simulink model "test_mdl_NI"  (R2018a)
settings: Solver=VariableStepAuto  StartTime=0.0  StopTime=10.0  RelTol=1e-3
(part 4 of 24)

== system test_mdl_NI/CAN_Signal/ABS_ESC/TesterPhysicalResABS_0x768 ==
  in : Inport
  TesterPhysicalResABS : Subsystem
  bus_creator : BusCreator  Inputs=1
  bus_selector : BusSelector  OutputSignals=TesterPhysicalResABS
  out_port : Outport
  wires:
  bus_creator/1 -> out_port/1  "TesterPhysicalResABS_0x768"
  TesterPhysicalResABS/1(out) -> bus_creator/1  "TesterPhysicalResABS"
  bus_selector/1 -> TesterPhysicalResABS/1(in)  "<TesterPhysicalResABS>"
  in/1 -> bus_selector/1

== system test_mdl_NI/CAN_Signal/ABS_ESC/TrailerBrakeData_0x412 ==
  in : Inport
  TrlrBrk_Pc_Rq : Subsystem
  VehPtch_An_Dsply : Subsystem
  VehRol_An_Dsply : Subsystem
  bus_creator : BusCreator  Inputs=3
  bus_selector : BusSelector  OutputSignals=TrlrBrk_Pc_Rq,VehPtch_An_Dsply,VehRol_An_Dsply
  out_port : Outport
  wires:
  bus_creator/1 -> out_port/1  "TrailerBrakeData_0x412"
  TrlrBrk_Pc_Rq/1(out) -> bus_creator/1  "TrlrBrk_Pc_Rq"
  VehPtch_An_Dsply/1(out) -> bus_creator/2  "VehPtch_An_Dsply"
  VehRol_An_Dsply/1(out) -> bus_creator/3  "VehRol_An_Dsply"
  bus_selector/1 -> TrlrBrk_Pc_Rq/1(in)  "<TrlrBrk_Pc_Rq>"
  bus_selector/2 -> VehPtch_An_Dsply/1(in)  "<VehPtch_An_Dsply>"
  bus_selector/3 -> VehRol_An_Dsply/1(in)  "<VehRol_An_Dsply>"
  in/1 -> bus_selector/1

== system test_mdl_NI/CAN_Signal/ABS_ESC/WheelData_0x216 ==
  in : Inport
  BrkObdData_No_Actl : Subsystem
  BrkObdIndex_No_Actl : Subsystem
  WhlDirFl_D_Actl : Subsystem
  WhlDirFr_D_Actl : Subsystem
  WhlDirRl_D_Actl : Subsystem
  WhlDirRr_D_Actl : Subsystem
  WhlRotatFl_No_Cnt : Subsystem
  WhlRotatFr_No_Cnt : Subsystem
  WhlRotatRl_No_Cnt : Subsystem
  WhlRotatRr_No_Cnt : Subsystem
  bus_creator : BusCreator  Inputs=10
  bus_selector : BusSelector  OutputSignals=WhlRotatFr_No_Cnt,WhlRotatFl_No_Cnt,WhlRotatRr_No_Cnt,WhlRotatRl_No_Cnt,WhlDirRl_D_Actl,WhlDirFr_D_Actl,WhlDirFl_D_Actl,WhlDirRr_D_Actl,BrkObdIndex_No_Actl,BrkObdData_No_Actl
  out_port : Outport
  wires:
  bus_creator/1 -> out_port/1  "WheelData_0x216"
  WhlRotatFr_No_Cnt/1(out) -> bus_creator/1  "WhlRotatFr_No_Cnt"
  WhlRotatFl_No_Cnt/1(out) -> bus_creator/2  "WhlRotatFl_No_Cnt"
  WhlRotatRr_No_Cnt/1(out) -> bus_creator/3  "WhlRotatRr_No_Cnt"
  WhlRotatRl_No_Cnt/1(out) -> bus_creator/4  "WhlRotatRl_No_Cnt"
  WhlDirRl_D_Actl/1(out) -> bus_creator/5  "WhlDirRl_D_Actl"
  WhlDirFr_D_Actl/1(out) -> bus_creator/6  "WhlDirFr_D_Actl"
  WhlDirFl_D_Actl/1(out) -> bus_creator/7  "WhlDirFl_D_Actl"
  WhlDirRr_D_Actl/1(out) -> bus_creator/8  "WhlDirRr_D_Actl"
  BrkObdIndex_No_Actl/1(out) -> bus_creator/9  "BrkObdIndex_No_Actl"
  BrkObdData_No_Actl/1(out) -> bus_creator/10  "BrkObdData_No_Actl"
  bus_selector/1 -> WhlRotatFr_No_Cnt/1(in)  "<WhlRotatFr_No_Cnt>"
  bus_selector/2 -> WhlRotatFl_No_Cnt/1(in)  "<WhlRotatFl_No_Cnt>"
  bus_selector/3 -> WhlRotatRr_No_Cnt/1(in)  "<WhlRotatRr_No_Cnt>"
  bus_selector/4 -> WhlRotatRl_No_Cnt/1(in)  "<WhlRotatRl_No_Cnt>"
  bus_selector/5 -> WhlDirRl_D_Actl/1(in)  "<WhlDirRl_D_Actl>"
  bus_selector/6 -> WhlDirFr_D_Actl/1(in)  "<WhlDirFr_D_Actl>"
  bus_selector/7 -> WhlDirFl_D_Actl/1(in)  "<WhlDirFl_D_Actl>"
  bus_selector/8 -> WhlDirRr_D_Actl/1(in)  "<WhlDirRr_D_Actl>"
  bus_selector/9 -> BrkObdIndex_No_Actl/1(in)  "<BrkObdIndex_No_Actl>"
  bus_selector/10 -> BrkObdData_No_Actl/1(in)  "<BrkObdData_No_Actl>"
  in/1 -> bus_selector/1

== system test_mdl_NI/CAN_Signal/ABS_ESC/WheelSpeed_0x217 ==
  in : Inport
  WhlFl_W_Meas : Subsystem
  WhlFr_W_Meas : Subsystem
  WhlRl_W_Meas : Subsystem
  WhlRr_W_Meas : Subsystem
  bus_creator : BusCreator  Inputs=4
  bus_selector : BusSelector  OutputSignals=WhlFl_W_Meas,WhlFr_W_Meas,WhlRl_W_Meas,WhlRr_W_Meas
  out_port : Outport
  wires:
  bus_creator/1 -> out_port/1  "WheelSpeed_0x217"
  WhlFl_W_Meas/1(out) -> bus_creator/1  "WhlFl_W_Meas"
  WhlFr_W_Meas/1(out) -> bus_creator/2  "WhlFr_W_Meas"
  WhlRl_W_Meas/1(out) -> bus_creator/3  "WhlRl_W_Meas"
  WhlRr_W_Meas/1(out) -> bus_creator/4  "WhlRr_W_Meas"
  bus_selector/1 -> WhlFl_W_Meas/1(in)  "<WhlFl_W_Meas>"
  bus_selector/2 -> WhlFr_W_Meas/1(in)  "<WhlFr_W_Meas>"
  bus_selector/3 -> WhlRl_W_Meas/1(in)  "<WhlRl_W_Meas>"
  bus_selector/4 -> WhlRr_W_Meas/1(in)  "<WhlRr_W_Meas>"
  in/1 -> bus_selector/1

== system test_mdl_NI/CAN_Signal/ADAS/ACCDATA ==
  in : Inport
  AccBrkDecel_B_Rq : Subsystem
  AccBrkPrchg_B_Rq : Subsystem
  AccBrkTot_A_Rq : Subsystem
  AccCancl_B_Rq : Subsystem
  AccPrpl_A_Rq : Subsystem
  AccPrpl_A_Rq1 : Subsystem
  AccStopStat_B_Rq : Subsystem
  CmbbEngTqMn_B_Rq : Subsystem
  bus_creator : BusCreator  Inputs=8
  bus_selector : BusSelector  OutputSignals=AccBrkPrchg_B_Rq,AccBrkDecel_B_Rq,AccStopStat_B_Rq,AccBrkTot_A_Rq,CmbbEngTqMn_B_Rq,AccCancl_B_Rq,AccPrpl_A_Rq,AccPrpl_A_Rq1
  out_port : Outport
  wires:
  bus_creator/1 -> out_port/1  "ACCDATA"
  AccBrkPrchg_B_Rq/1(out) -> bus_creator/1  "AccBrkPrchg_B_Rq"
  AccBrkDecel_B_Rq/1(out) -> bus_creator/2  "AccBrkDecel_B_Rq"
  AccStopStat_B_Rq/1(out) -> bus_creator/3  "AccStopStat_B_Rq"
  AccBrkTot_A_Rq/1(out) -> bus_creator/4  "AccBrkTot_A_Rq"
  CmbbEngTqMn_B_Rq/1(out) -> bus_creator/5  "CmbbEngTqMn_B_Rq"
  AccCancl_B_Rq/1(out) -> bus_creator/6  "AccCancl_B_Rq"
  AccPrpl_A_Rq/1(out) -> bus_creator/7  "AccPrpl_A_Rq"
  AccPrpl_A_Rq1/1(out) -> bus_creator/8  "AccPrpl_A_Rq1"
  bus_selector/1 -> AccBrkPrchg_B_Rq/1(in)  "<AccBrkPrchg_B_Rq>"
  bus_selector/2 -> AccBrkDecel_B_Rq/1(in)  "<AccBrkDecel_B_Rq>"
  bus_selector/3 -> AccStopStat_B_Rq/1(in)  "<AccStopStat_B_Rq>"
  bus_selector/4 -> AccBrkTot_A_Rq/1(in)  "<AccBrkTot_A_Rq>"
  bus_selector/5 -> CmbbEngTqMn_B_Rq/1(in)  "<CmbbEngTqMn_B_Rq>"
  bus_selector/6 -> AccCancl_B_Rq/1(in)  "<AccCancl_B_Rq>"
  bus_selector/7 -> AccPrpl_A_Rq/1(in)  "<AccPrpl_A_Rq>"
  bus_selector/8 -> AccPrpl_A_Rq1/1(in)  "<AccPrpl_A_Rq1>"
  in/1 -> bus_selector/1

== system test_mdl_NI/CAN_Signal/ADAS/ACCDATA_2 ==
  in : Inport
  CmbbBaSens_D_Rq : Subsystem
  CmbbBrkDecel_A_Rq : Subsystem
  CmbbBrkDecel_B_Rq : Subsystem
  CmbbBrkPrchg_D_Rq : Subsystem
  bus_creator : BusCreator  Inputs=4
  bus_selector : BusSelector  OutputSignals=CmbbBrkPrchg_D_Rq,CmbbBrkDecel_A_Rq,CmbbBaSens_D_Rq,CmbbBrkDecel_B_Rq
  out_port : Outport
  wires:
  bus_creator/1 -> out_port/1  "ACCDATA_2"
  CmbbBrkPrchg_D_Rq/1(out) -> bus_creator/1  "CmbbBrkPrchg_D_Rq"
  CmbbBrkDecel_A_Rq/1(out) -> bus_creator/2  "CmbbBrkDecel_A_Rq"
  CmbbBaSens_D_Rq/1(out) -> bus_creator/3  "CmbbBaSens_D_Rq"
  CmbbBrkDecel_B_Rq/1(out) -> bus_creator/4  "CmbbBrkDecel_B_Rq"
  bus_selector/1 -> CmbbBrkPrchg_D_Rq/1(in)  "<CmbbBrkPrchg_D_Rq>"
  bus_selector/2 -> CmbbBrkDecel_A_Rq/1(in)  "<CmbbBrkDecel_A_Rq>"
  bus_selector/3 -> CmbbBaSens_D_Rq/1(in)  "<CmbbBaSens_D_Rq>"
  bus_selector/4 -> CmbbBrkDecel_B_Rq/1(in)  "<CmbbBrkDecel_B_Rq>"
  in/1 -> bus_selector/1

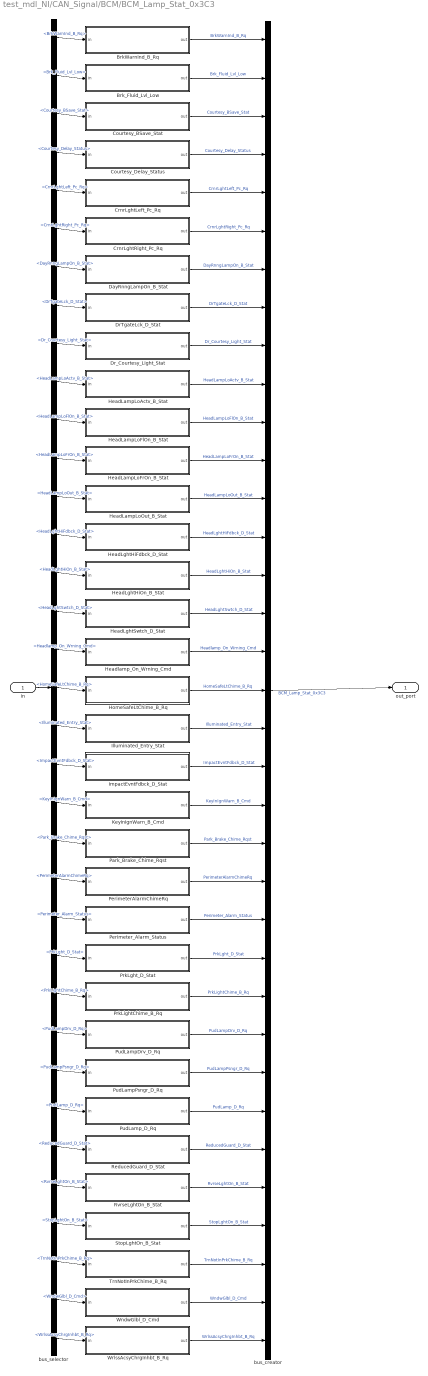
== system test_mdl_NI/CAN_Signal/BCM/BCM_Lamp_Stat_0x3C3 ==
  in : Inport
  BrkWarnInd_B_Rq : Subsystem
  Brk_Fluid_Lvl_Low : Subsystem
  Courtesy_BSave_Stat : Subsystem
  Courtesy_Delay_Status : Subsystem
  CrnrLghtLeft_Pc_Rq : Subsystem
  CrnrLghtRight_Pc_Rq : Subsystem
  DayRnngLampOn_B_Stat : Subsystem
  DrTgateLck_D_Stat : Subsystem
  Dr_Courtesy_Light_Stat : Subsystem
  HeadLampLoActv_B_Stat : Subsystem
  HeadLampLoFlOn_B_Stat : Subsystem
  HeadLampLoFrOn_B_Stat : Subsystem
  HeadLampLoOut_B_Stat : Subsystem
  HeadLghtHiFdbck_D_Stat : Subsystem
  HeadLghtHiOn_B_Stat : Subsystem
  HeadLghtSwtch_D_Stat : Subsystem
  Headlamp_On_Wrning_Cmd : Subsystem
  HomeSafeLtChime_B_Rq : Subsystem
  Illuminated_Entry_Stat : Subsystem
  ImpactEvntFdbck_D_Stat : Subsystem
  KeyInIgnWarn_B_Cmd : Subsystem
  Park_Brake_Chime_Rqst : Subsystem
  PerimeterAlarmChimeRq : Subsystem
  Perimeter_Alarm_Status : Subsystem
  PrkLght_D_Stat : Subsystem
  PrkLightChime_B_Rq : Subsystem
  PudLampDrv_D_Rq : Subsystem
  PudLampPsngr_D_Rq : Subsystem
  PudLamp_D_Rq : Subsystem
  ReducedGuard_D_Stat : Subsystem
  RvrseLghtOn_B_Stat : Subsystem
  StopLghtOn_B_Stat : Subsystem
  TrnNotInPrkChime_B_Rq : Subsystem
  WndwGlbl_D_Cmd : Subsystem
  WrlssAcsyChrgInhbt_B_Rq : Subsystem
  bus_creator : BusCreator  Inputs=35
  bus_selector : BusSelector  OutputSignals=BrkWarnInd_B_Rq,Brk_Fluid_Lvl_Low,Courtesy_BSave_Stat,Courtesy_Delay_Status,CrnrLghtLeft_Pc_Rq,CrnrLghtRight_Pc_Rq,DayRnngLampOn_B_Stat,DrTgateLck_D_Stat,Dr_Courtesy_Light_Stat,HeadLampLoActv_B_Stat,HeadLampLoFlOn_B_Stat,HeadLampLoFrOn_B_Stat,HeadLampLoOut_B_Stat,HeadLghtHiFdbck_D_Stat,HeadLghtHiOn_B_Stat,HeadLghtSwtch_D_Stat,Headlamp_On_Wrning_Cmd,HomeSafeLtChime_B_Rq,Illuminated_Entry_Stat,ImpactEvntFdbck_D_Stat,KeyInIgnWarn_B_Cmd,Park_Brake_Chime_Rqst,PerimeterAlarmChimeRq,Perimeter_Alarm_Status,PrkLght_D_Stat,PrkLightChime_B_Rq,PudLampDrv_D_Rq,PudLampPsngr_D_Rq,PudLamp_D_Rq,ReducedGuard_D_Stat,RvrseLghtOn_B_Stat,StopLghtOn_B_Stat,TrnNotInPrkChime_B_Rq,WndwGlbl_D_Cmd,WrlssAcsyChrgInhbt_B_Rq
  out_port : Outport
  wires:
  bus_creator/1 -> out_port/1  "BCM_Lamp_Stat_0x3C3"
  BrkWarnInd_B_Rq/1(out) -> bus_creator/1  "BrkWarnInd_B_Rq"
  Brk_Fluid_Lvl_Low/1(out) -> bus_creator/2  "Brk_Fluid_Lvl_Low"
  Courtesy_BSave_Stat/1(out) -> bus_creator/3  "Courtesy_BSave_Stat"
  Courtesy_Delay_Status/1(out) -> bus_creator/4  "Courtesy_Delay_Status"
  CrnrLghtLeft_Pc_Rq/1(out) -> bus_creator/5  "CrnrLghtLeft_Pc_Rq"
  CrnrLghtRight_Pc_Rq/1(out) -> bus_creator/6  "CrnrLghtRight_Pc_Rq"
  DayRnngLampOn_B_Stat/1(out) -> bus_creator/7  "DayRnngLampOn_B_Stat"
  DrTgateLck_D_Stat/1(out) -> bus_creator/8  "DrTgateLck_D_Stat"
  Dr_Courtesy_Light_Stat/1(out) -> bus_creator/9  "Dr_Courtesy_Light_Stat"
  HeadLampLoActv_B_Stat/1(out) -> bus_creator/10  "HeadLampLoActv_B_Stat"
  HeadLampLoFlOn_B_Stat/1(out) -> bus_creator/11  "HeadLampLoFlOn_B_Stat"
  HeadLampLoFrOn_B_Stat/1(out) -> bus_creator/12  "HeadLampLoFrOn_B_Stat"
  HeadLampLoOut_B_Stat/1(out) -> bus_creator/13  "HeadLampLoOut_B_Stat"
  HeadLghtHiFdbck_D_Stat/1(out) -> bus_creator/14  "HeadLghtHiFdbck_D_Stat"
  HeadLghtHiOn_B_Stat/1(out) -> bus_creator/15  "HeadLghtHiOn_B_Stat"
  HeadLghtSwtch_D_Stat/1(out) -> bus_creator/16  "HeadLghtSwtch_D_Stat"
  Headlamp_On_Wrning_Cmd/1(out) -> bus_creator/17  "Headlamp_On_Wrning_Cmd"
  HomeSafeLtChime_B_Rq/1(out) -> bus_creator/18  "HomeSafeLtChime_B_Rq"
  Illuminated_Entry_Stat/1(out) -> bus_creator/19  "Illuminated_Entry_Stat"
  ImpactEvntFdbck_D_Stat/1(out) -> bus_creator/20  "ImpactEvntFdbck_D_Stat"
  KeyInIgnWarn_B_Cmd/1(out) -> bus_creator/21  "KeyInIgnWarn_B_Cmd"
  Park_Brake_Chime_Rqst/1(out) -> bus_creator/22  "Park_Brake_Chime_Rqst"
  PerimeterAlarmChimeRq/1(out) -> bus_creator/23  "PerimeterAlarmChimeRq"
  Perimeter_Alarm_Status/1(out) -> bus_creator/24  "Perimeter_Alarm_Status"
  PrkLght_D_Stat/1(out) -> bus_creator/25  "PrkLght_D_Stat"
  PrkLightChime_B_Rq/1(out) -> bus_creator/26  "PrkLightChime_B_Rq"
  PudLampDrv_D_Rq/1(out) -> bus_creator/27  "PudLampDrv_D_Rq"
  PudLampPsngr_D_Rq/1(out) -> bus_creator/28  "PudLampPsngr_D_Rq"
  PudLamp_D_Rq/1(out) -> bus_creator/29  "PudLamp_D_Rq"
  ReducedGuard_D_Stat/1(out) -> bus_creator/30  "ReducedGuard_D_Stat"
  RvrseLghtOn_B_Stat/1(out) -> bus_creator/31  "RvrseLghtOn_B_Stat"
  StopLghtOn_B_Stat/1(out) -> bus_creator/32  "StopLghtOn_B_Stat"
  TrnNotInPrkChime_B_Rq/1(out) -> bus_creator/33  "TrnNotInPrkChime_B_Rq"
  WndwGlbl_D_Cmd/1(out) -> bus_creator/34  "WndwGlbl_D_Cmd"
  WrlssAcsyChrgInhbt_B_Rq/1(out) -> bus_creator/35  "WrlssAcsyChrgInhbt_B_Rq"
  bus_selector/1 -> BrkWarnInd_B_Rq/1(in)  "<BrkWarnInd_B_Rq>"
  bus_selector/2 -> Brk_Fluid_Lvl_Low/1(in)  "<Brk_Fluid_Lvl_Low>"
  bus_selector/3 -> Courtesy_BSave_Stat/1(in)  "<Courtesy_BSave_Stat>"
  bus_selector/4 -> Courtesy_Delay_Status/1(in)  "<Courtesy_Delay_Status>"
  bus_selector/5 -> CrnrLghtLeft_Pc_Rq/1(in)  "<CrnrLghtLeft_Pc_Rq>"
  bus_selector/6 -> CrnrLghtRight_Pc_Rq/1(in)  "<CrnrLghtRight_Pc_Rq>"
  bus_selector/7 -> DayRnngLampOn_B_Stat/1(in)  "<DayRnngLampOn_B_Stat>"
  bus_selector/8 -> DrTgateLck_D_Stat/1(in)  "<DrTgateLck_D_Stat>"
  bus_selector/9 -> Dr_Courtesy_Light_Stat/1(in)  "<Dr_Courtesy_Light_Stat>"
  bus_selector/10 -> HeadLampLoActv_B_Stat/1(in)  "<HeadLampLoActv_B_Stat>"
  bus_selector/11 -> HeadLampLoFlOn_B_Stat/1(in)  "<HeadLampLoFlOn_B_Stat>"
  bus_selector/12 -> HeadLampLoFrOn_B_Stat/1(in)  "<HeadLampLoFrOn_B_Stat>"
  bus_selector/13 -> HeadLampLoOut_B_Stat/1(in)  "<HeadLampLoOut_B_Stat>"
  bus_selector/14 -> HeadLghtHiFdbck_D_Stat/1(in)  "<HeadLghtHiFdbck_D_Stat>"
  bus_selector/15 -> HeadLghtHiOn_B_Stat/1(in)  "<HeadLghtHiOn_B_Stat>"
  bus_selector/16 -> HeadLghtSwtch_D_Stat/1(in)  "<HeadLghtSwtch_D_Stat>"
  bus_selector/17 -> Headlamp_On_Wrning_Cmd/1(in)  "<Headlamp_On_Wrning_Cmd>"
  bus_selector/18 -> HomeSafeLtChime_B_Rq/1(in)  "<HomeSafeLtChime_B_Rq>"
  bus_selector/19 -> Illuminated_Entry_Stat/1(in)  "<Illuminated_Entry_Stat>"
  bus_selector/20 -> ImpactEvntFdbck_D_Stat/1(in)  "<ImpactEvntFdbck_D_Stat>"
  bus_selector/21 -> KeyInIgnWarn_B_Cmd/1(in)  "<KeyInIgnWarn_B_Cmd>"
  bus_selector/22 -> Park_Brake_Chime_Rqst/1(in)  "<Park_Brake_Chime_Rqst>"
  bus_selector/23 -> PerimeterAlarmChimeRq/1(in)  "<PerimeterAlarmChimeRq>"
  bus_selector/24 -> Perimeter_Alarm_Status/1(in)  "<Perimeter_Alarm_Status>"
  bus_selector/25 -> PrkLght_D_Stat/1(in)  "<PrkLght_D_Stat>"
  bus_selector/26 -> PrkLightChime_B_Rq/1(in)  "<PrkLightChime_B_Rq>"
  bus_selector/27 -> PudLampDrv_D_Rq/1(in)  "<PudLampDrv_D_Rq>"
  bus_selector/28 -> PudLampPsngr_D_Rq/1(in)  "<PudLampPsngr_D_Rq>"
  bus_selector/29 -> PudLamp_D_Rq/1(in)  "<PudLamp_D_Rq>"
  bus_selector/30 -> ReducedGuard_D_Stat/1(in)  "<ReducedGuard_D_Stat>"
  bus_selector/31 -> RvrseLghtOn_B_Stat/1(in)  "<RvrseLghtOn_B_Stat>"
  bus_selector/32 -> StopLghtOn_B_Stat/1(in)  "<StopLghtOn_B_Stat>"
  bus_selector/33 -> TrnNotInPrkChime_B_Rq/1(in)  "<TrnNotInPrkChime_B_Rq>"
  bus_selector/34 -> WndwGlbl_D_Cmd/1(in)  "<WndwGlbl_D_Cmd>"
  bus_selector/35 -> WrlssAcsyChrgInhbt_B_Rq/1(in)  "<WrlssAcsyChrgInhbt_B_Rq>"
  in/1 -> bus_selector/1

== system test_mdl_NI/CAN_Signal/BCM/Battery_Mgmt_24V_0x42E ==
  in : Inport
  BattULo24Soc_Pc_Actl : Subsystem
  BattULo24State_D_Qlty : Subsystem
  BattULo24_Ah_DeltaRide : Subsystem
  BattULo24_B_Falt : Subsystem
  BattULo24_I_Actl : Subsystem
  bus_creator : BusCreator  Inputs=5
  bus_selector : BusSelector  OutputSignals=BattULo24_Ah_DeltaRide,BattULo24_B_Falt,BattULo24_I_Actl,BattULo24State_D_Qlty,BattULo24Soc_Pc_Actl
  out_port : Outport
  wires:
  bus_creator/1 -> out_port/1  "Battery_Mgmt_24V_0x42E"
  BattULo24_Ah_DeltaRide/1(out) -> bus_creator/1  "BattULo24_Ah_DeltaRide"
  BattULo24_B_Falt/1(out) -> bus_creator/2  "BattULo24_B_Falt"
  BattULo24_I_Actl/1(out) -> bus_creator/3  "BattULo24_I_Actl"
  BattULo24State_D_Qlty/1(out) -> bus_creator/4  "BattULo24State_D_Qlty"
  BattULo24Soc_Pc_Actl/1(out) -> bus_creator/5  "BattULo24Soc_Pc_Actl"
  bus_selector/1 -> BattULo24_Ah_DeltaRide/1(in)  "<BattULo24_Ah_DeltaRide>"
  bus_selector/2 -> BattULo24_B_Falt/1(in)  "<BattULo24_B_Falt>"
  bus_selector/3 -> BattULo24_I_Actl/1(in)  "<BattULo24_I_Actl>"
  bus_selector/4 -> BattULo24State_D_Qlty/1(in)  "<BattULo24State_D_Qlty>"
  bus_selector/5 -> BattULo24Soc_Pc_Actl/1(in)  "<BattULo24Soc_Pc_Actl>"
  in/1 -> bus_selector/1

== system test_mdl_NI/CAN_Signal/BCM/Battery_Mgmt_2_0x42C ==
  in : Inport
  BattULoChrg_D_Rq : Subsystem
  BattULoSrvc_T_Actl : Subsystem
  Batt_Crit_SoC_B : Subsystem
  Batt_Lo_SoC_B : Subsystem
  ChargeMode : Subsystem
  EngStrtInhbt_B_RqBatt : Subsystem
  IdleSpeedIncrease_El : Subsystem
  PeriodicElLoad_B_Stat : Subsystem
  PwSysULoFalt_D_Stat : Subsystem
  Shed_Drain_Eng_Off_B : Subsystem
  Shed_Feature_Group_ID : Subsystem
  Shed_Level_Req : Subsystem
  Shed_T_Eng_Off_B : Subsystem
  ULoRgenTestMde_B_Rq : Subsystem
  bus_creator : BusCreator  Inputs=14
  bus_selector : BusSelector  OutputSignals=BattULoChrg_D_Rq,BattULoSrvc_T_Actl,Batt_Crit_SoC_B,Batt_Lo_SoC_B,ChargeMode,EngStrtInhbt_B_RqBatt,IdleSpeedIncrease_El,PeriodicElLoad_B_Stat,PwSysULoFalt_D_Stat,Shed_Drain_Eng_Off_B,Shed_Feature_Group_ID,Shed_Level_Req,Shed_T_Eng_Off_B,ULoRgenTestMde_B_Rq
  out_port : Outport
  wires:
  bus_creator/1 -> out_port/1  "Battery_Mgmt_2_0x42C"
  BattULoChrg_D_Rq/1(out) -> bus_creator/1  "BattULoChrg_D_Rq"
  BattULoSrvc_T_Actl/1(out) -> bus_creator/2  "BattULoSrvc_T_Actl"
  Batt_Crit_SoC_B/1(out) -> bus_creator/3  "Batt_Crit_SoC_B"
  Batt_Lo_SoC_B/1(out) -> bus_creator/4  "Batt_Lo_SoC_B"
  ChargeMode/1(out) -> bus_creator/5  "ChargeMode"
  EngStrtInhbt_B_RqBatt/1(out) -> bus_creator/6  "EngStrtInhbt_B_RqBatt"
  IdleSpeedIncrease_El/1(out) -> bus_creator/7  "IdleSpeedIncrease_El"
  PeriodicElLoad_B_Stat/1(out) -> bus_creator/8  "PeriodicElLoad_B_Stat"
  PwSysULoFalt_D_Stat/1(out) -> bus_creator/9  "PwSysULoFalt_D_Stat"
  Shed_Drain_Eng_Off_B/1(out) -> bus_creator/10  "Shed_Drain_Eng_Off_B"
  Shed_Feature_Group_ID/1(out) -> bus_creator/11  "Shed_Feature_Group_ID"
  Shed_Level_Req/1(out) -> bus_creator/12  "Shed_Level_Req"
  Shed_T_Eng_Off_B/1(out) -> bus_creator/13  "Shed_T_Eng_Off_B"
  ULoRgenTestMde_B_Rq/1(out) -> bus_creator/14  "ULoRgenTestMde_B_Rq"
  bus_selector/1 -> BattULoChrg_D_Rq/1(in)  "<BattULoChrg_D_Rq>"
  bus_selector/2 -> BattULoSrvc_T_Actl/1(in)  "<BattULoSrvc_T_Actl>"
  bus_selector/3 -> Batt_Crit_SoC_B/1(in)  "<Batt_Crit_SoC_B>"
  bus_selector/4 -> Batt_Lo_SoC_B/1(in)  "<Batt_Lo_SoC_B>"
  bus_selector/5 -> ChargeMode/1(in)  "<ChargeMode>"
  bus_selector/6 -> EngStrtInhbt_B_RqBatt/1(in)  "<EngStrtInhbt_B_RqBatt>"
  bus_selector/7 -> IdleSpeedIncrease_El/1(in)  "<IdleSpeedIncrease_El>"
  bus_selector/8 -> PeriodicElLoad_B_Stat/1(in)  "<PeriodicElLoad_B_Stat>"
  bus_selector/9 -> PwSysULoFalt_D_Stat/1(in)  "<PwSysULoFalt_D_Stat>"
  bus_selector/10 -> Shed_Drain_Eng_Off_B/1(in)  "<Shed_Drain_Eng_Off_B>"
  bus_selector/11 -> Shed_Feature_Group_ID/1(in)  "<Shed_Feature_Group_ID>"
  bus_selector/12 -> Shed_Level_Req/1(in)  "<Shed_Level_Req>"
  bus_selector/13 -> Shed_T_Eng_Off_B/1(in)  "<Shed_T_Eng_Off_B>"
  bus_selector/14 -> ULoRgenTestMde_B_Rq/1(in)  "<ULoRgenTestMde_B_Rq>"
  in/1 -> bus_selector/1

== system test_mdl_NI/CAN_Signal/BCM/Battery_Mgmt_3_0x43C ==
  in : Inport
  BSBattQCapAh : Subsystem
  BSBattQDeltaRideAh : Subsystem
  BSBattSOC : Subsystem
  BSFault : Subsystem
  BattULo2_Te_Actl : Subsystem
  BattULoChrg_URate_RqMx : Subsystem
  BattULoChrg_U_RqMn : Subsystem
  BattULoChrg_U_RqMx : Subsystem
  BattULoState_D_Qlty : Subsystem
  bus_creator : BusCreator  Inputs=9
  bus_selector : BusSelector  OutputSignals=BSFault,BSBattQDeltaRideAh,BSBattSOC,BattULo2_Te_Actl,BSBattQCapAh,BattULoState_D_Qlty,BattULoChrg_U_RqMn,BattULoChrg_U_RqMx,BattULoChrg_URate_RqMx
  out_port : Outport
  wires:
  bus_creator/1 -> out_port/1  "Battery_Mgmt_3_0x43C"
  BSFault/1(out) -> bus_creator/1  "BSFault"
  BSBattQDeltaRideAh/1(out) -> bus_creator/2  "BSBattQDeltaRideAh"
  BSBattSOC/1(out) -> bus_creator/3  "BSBattSOC"
  BattULo2_Te_Actl/1(out) -> bus_creator/4  "BattULo2_Te_Actl"
  BSBattQCapAh/1(out) -> bus_creator/5  "BSBattQCapAh"
  BattULoState_D_Qlty/1(out) -> bus_creator/6  "BattULoState_D_Qlty"
  BattULoChrg_U_RqMn/1(out) -> bus_creator/7  "BattULoChrg_U_RqMn"
  BattULoChrg_U_RqMx/1(out) -> bus_creator/8  "BattULoChrg_U_RqMx"
  BattULoChrg_URate_RqMx/1(out) -> bus_creator/9  "BattULoChrg_URate_RqMx"
  bus_selector/1 -> BSFault/1(in)  "<BSFault>"
  bus_selector/2 -> BSBattQDeltaRideAh/1(in)  "<BSBattQDeltaRideAh>"
  bus_selector/3 -> BSBattSOC/1(in)  "<BSBattSOC>"
  bus_selector/4 -> BattULo2_Te_Actl/1(in)  "<BattULo2_Te_Actl>"
  bus_selector/5 -> BSBattQCapAh/1(in)  "<BSBattQCapAh>"
  bus_selector/6 -> BattULoState_D_Qlty/1(in)  "<BattULoState_D_Qlty>"
  bus_selector/7 -> BattULoChrg_U_RqMn/1(in)  "<BattULoChrg_U_RqMn>"
  bus_selector/8 -> BattULoChrg_U_RqMx/1(in)  "<BattULoChrg_U_RqMx>"
  bus_selector/9 -> BattULoChrg_URate_RqMx/1(in)  "<BattULoChrg_URate_RqMx>"
  in/1 -> bus_selector/1

== system test_mdl_NI/CAN_Signal/BCM/Battery_Mgmt_4_0x42B ==
  in : Inport
  BattULoAuxSoc_Pc_Actl : Subsystem
  BattULoAux_B_Falt : Subsystem
  BattULoAux_D_Qlty : Subsystem
  BattULoAux_I_Actl : Subsystem
  BattULoAux_U_Actl : Subsystem
  BattULoCrnkBelt_U_Pred : Subsystem
  BattULoCrnkStrt_U_Pred : Subsystem
  bus_creator : BusCreator  Inputs=7
  bus_selector : BusSelector  OutputSignals=BattULoAux_U_Actl,BattULoAuxSoc_Pc_Actl,BattULoAux_B_Falt,BattULoAux_I_Actl,BattULoAux_D_Qlty,BattULoCrnkBelt_U_Pred,BattULoCrnkStrt_U_Pred
  out_port : Outport
  wires:
  bus_creator/1 -> out_port/1  "Battery_Mgmt_4_0x42B"
  BattULoAux_U_Actl/1(out) -> bus_creator/1  "BattULoAux_U_Actl"
  BattULoAuxSoc_Pc_Actl/1(out) -> bus_creator/2  "BattULoAuxSoc_Pc_Actl"
  BattULoAux_B_Falt/1(out) -> bus_creator/3  "BattULoAux_B_Falt"
  BattULoAux_I_Actl/1(out) -> bus_creator/4  "BattULoAux_I_Actl"
  BattULoAux_D_Qlty/1(out) -> bus_creator/5  "BattULoAux_D_Qlty"
  BattULoCrnkBelt_U_Pred/1(out) -> bus_creator/6  "BattULoCrnkBelt_U_Pred"
  BattULoCrnkStrt_U_Pred/1(out) -> bus_creator/7  "BattULoCrnkStrt_U_Pred"
  bus_selector/1 -> BattULoAux_U_Actl/1(in)  "<BattULoAux_U_Actl>"
  bus_selector/2 -> BattULoAuxSoc_Pc_Actl/1(in)  "<BattULoAuxSoc_Pc_Actl>"
  bus_selector/3 -> BattULoAux_B_Falt/1(in)  "<BattULoAux_B_Falt>"
  bus_selector/4 -> BattULoAux_I_Actl/1(in)  "<BattULoAux_I_Actl>"
  bus_selector/5 -> BattULoAux_D_Qlty/1(in)  "<BattULoAux_D_Qlty>"
  bus_selector/6 -> BattULoCrnkBelt_U_Pred/1(in)  "<BattULoCrnkBelt_U_Pred>"
  bus_selector/7 -> BattULoCrnkStrt_U_Pred/1(in)  "<BattULoCrnkStrt_U_Pred>"
  in/1 -> bus_selector/1

== system test_mdl_NI/CAN_Signal/BCM/BodyInfo_3_0x3B3 ==
  in : Inport
  Backlit_LED_Status : Subsystem
  BodySrvcRqd_B_Rq : Subsystem
  CrashEvnt_D_Stat : Subsystem
  Day_Night_Status : Subsystem
  Delay_Accy : Subsystem
  DimmingLvlEvnt_No_Actl : Subsystem
  Dimming_Lvl : Subsystem
  DrStatDrvErrCnt_B_Stat : Subsystem
  DrStatDrv_B_Actl : Subsystem
  DrStatHood_B_Actl : Subsystem
  DrStatInnrTgate_B_Actl : Subsystem
  DrStatPsngr_B_Actl : Subsystem
  DrStatRl_B_Actl : Subsystem
  DrStatRr_B_Actl : Subsystem
  DrStatTgate_B_Actl : Subsystem
  FogLghtFrontOn_B_Stat : Subsystem
  FogLghtRearOn_B_Stat : Subsystem
  FuelPmpInhbt_B_Stat : Subsystem
  IgnKeyType_D_Actl : Subsystem
  Ignition_Status : Subsystem
  Key_In_Ignition_Stat : Subsystem
  LifeCycMde_D_Actl : Subsystem
  Litval : Subsystem
  Parklamp_Status : Subsystem
  PrkBrkActv_B_Actl : Subsystem
  Remote_Start_Status : Subsystem
  TurnLghtLeftOn_B_Stat : Subsystem
  TurnLghtLeft_D_Rq : Subsystem
  TurnLghtRightOn_B_Stat : Subsystem
  TurnLghtRight_D_Rq : Subsystem
  ValetMode_D_Mem : Subsystem
  bus_creator : BusCreator  Inputs=31
  bus_selector : BusSelector  OutputSignals=Ignition_Status,Parklamp_Status,FogLghtRearOn_B_Stat,DrStatTgate_B_Actl,Day_Night_Status,Remote_Start_Status,Key_In_Ignition_Stat,BodySrvcRqd_B_Rq,TurnLghtLeft_D_Rq,Backlit_LED_Status,DrStatDrvErrCnt_B_Stat,DimmingLvlEvnt_No_Actl,ValetMode_D_Mem,Dimming_Lvl,IgnKeyType_D_Actl,TurnLghtRightOn_B_Stat,CrashEvnt_D_Stat,FuelPmpInhbt_B_Stat,Litval,PrkBrkActv_B_Actl,TurnLghtLeftOn_B_Stat,LifeCycMde_D_Actl,DrStatRr_B_Actl,DrStatRl_B_Actl,TurnLghtRight_D_Rq,DrStatDrv_B_Actl,DrStatPsngr_B_Actl,DrStatHood_B_Actl,DrStatInnrTgate_B_Actl,Delay_Accy,FogLghtFrontOn_B_Stat
  out_port : Outport
  wires:
  bus_creator/1 -> out_port/1  "BodyInfo_3_0x3B3"
  Ignition_Status/1(out) -> bus_creator/1  "Ignition_Status"
  Parklamp_Status/1(out) -> bus_creator/2  "Parklamp_Status"
  FogLghtRearOn_B_Stat/1(out) -> bus_creator/3  "FogLghtRearOn_B_Stat"
  DrStatTgate_B_Actl/1(out) -> bus_creator/4  "DrStatTgate_B_Actl"
  Day_Night_Status/1(out) -> bus_creator/5  "Day_Night_Status"
  Remote_Start_Status/1(out) -> bus_creator/6  "Remote_Start_Status"
  Key_In_Ignition_Stat/1(out) -> bus_creator/7  "Key_In_Ignition_Stat"
  BodySrvcRqd_B_Rq/1(out) -> bus_creator/8  "BodySrvcRqd_B_Rq"
  TurnLghtLeft_D_Rq/1(out) -> bus_creator/9  "TurnLghtLeft_D_Rq"
  Backlit_LED_Status/1(out) -> bus_creator/10  "Backlit_LED_Status"
  DrStatDrvErrCnt_B_Stat/1(out) -> bus_creator/11  "DrStatDrvErrCnt_B_Stat"
  DimmingLvlEvnt_No_Actl/1(out) -> bus_creator/12  "DimmingLvlEvnt_No_Actl"
  ValetMode_D_Mem/1(out) -> bus_creator/13  "ValetMode_D_Mem"
  Dimming_Lvl/1(out) -> bus_creator/14  "Dimming_Lvl"
  IgnKeyType_D_Actl/1(out) -> bus_creator/15  "IgnKeyType_D_Actl"
  TurnLghtRightOn_B_Stat/1(out) -> bus_creator/16  "TurnLghtRightOn_B_Stat"
  CrashEvnt_D_Stat/1(out) -> bus_creator/17  "CrashEvnt_D_Stat"
  FuelPmpInhbt_B_Stat/1(out) -> bus_creator/18  "FuelPmpInhbt_B_Stat"
  Litval/1(out) -> bus_creator/19  "Litval"
  PrkBrkActv_B_Actl/1(out) -> bus_creator/20  "PrkBrkActv_B_Actl"
  TurnLghtLeftOn_B_Stat/1(out) -> bus_creator/21  "TurnLghtLeftOn_B_Stat"
  LifeCycMde_D_Actl/1(out) -> bus_creator/22  "LifeCycMde_D_Actl"
  DrStatRr_B_Actl/1(out) -> bus_creator/23  "DrStatRr_B_Actl"
  DrStatRl_B_Actl/1(out) -> bus_creator/24  "DrStatRl_B_Actl"
  TurnLghtRight_D_Rq/1(out) -> bus_creator/25  "TurnLghtRight_D_Rq"
  DrStatDrv_B_Actl/1(out) -> bus_creator/26  "DrStatDrv_B_Actl"
  DrStatPsngr_B_Actl/1(out) -> bus_creator/27  "DrStatPsngr_B_Actl"
  DrStatHood_B_Actl/1(out) -> bus_creator/28  "DrStatHood_B_Actl"
  DrStatInnrTgate_B_Actl/1(out) -> bus_creator/29  "DrStatInnrTgate_B_Actl"
  Delay_Accy/1(out) -> bus_creator/30  "Delay_Accy"
  FogLghtFrontOn_B_Stat/1(out) -> bus_creator/31  "FogLghtFrontOn_B_Stat"
  bus_selector/1 -> Ignition_Status/1(in)  "<Ignition_Status>"
  bus_selector/2 -> Parklamp_Status/1(in)  "<Parklamp_Status>"
  bus_selector/3 -> FogLghtRearOn_B_Stat/1(in)  "<FogLghtRearOn_B_Stat>"
  bus_selector/4 -> DrStatTgate_B_Actl/1(in)  "<DrStatTgate_B_Actl>"
  bus_selector/5 -> Day_Night_Status/1(in)  "<Day_Night_Status>"
  bus_selector/6 -> Remote_Start_Status/1(in)  "<Remote_Start_Status>"
  bus_selector/7 -> Key_In_Ignition_Stat/1(in)  "<Key_In_Ignition_Stat>"
  bus_selector/8 -> BodySrvcRqd_B_Rq/1(in)  "<BodySrvcRqd_B_Rq>"
  bus_selector/9 -> TurnLghtLeft_D_Rq/1(in)  "<TurnLghtLeft_D_Rq>"
  bus_selector/10 -> Backlit_LED_Status/1(in)  "<Backlit_LED_Status>"
  bus_selector/11 -> DrStatDrvErrCnt_B_Stat/1(in)  "<DrStatDrvErrCnt_B_Stat>"
  bus_selector/12 -> DimmingLvlEvnt_No_Actl/1(in)  "<DimmingLvlEvnt_No_Actl>"
  bus_selector/13 -> ValetMode_D_Mem/1(in)  "<ValetMode_D_Mem>"
  bus_selector/14 -> Dimming_Lvl/1(in)  "<Dimming_Lvl>"
  bus_selector/15 -> IgnKeyType_D_Actl/1(in)  "<IgnKeyType_D_Actl>"
  bus_selector/16 -> TurnLghtRightOn_B_Stat/1(in)  "<TurnLghtRightOn_B_Stat>"
  bus_selector/17 -> CrashEvnt_D_Stat/1(in)  "<CrashEvnt_D_Stat>"
  bus_selector/18 -> FuelPmpInhbt_B_Stat/1(in)  "<FuelPmpInhbt_B_Stat>"
  bus_selector/19 -> Litval/1(in)  "<Litval>"
  bus_selector/20 -> PrkBrkActv_B_Actl/1(in)  "<PrkBrkActv_B_Actl>"
  bus_selector/21 -> TurnLghtLeftOn_B_Stat/1(in)  "<TurnLghtLeftOn_B_Stat>"
  bus_selector/22 -> LifeCycMde_D_Actl/1(in)  "<LifeCycMde_D_Actl>"
  bus_selector/23 -> DrStatRr_B_Actl/1(in)  "<DrStatRr_B_Actl>"
  bus_selector/24 -> DrStatRl_B_Actl/1(in)  "<DrStatRl_B_Actl>"
  bus_selector/25 -> TurnLghtRight_D_Rq/1(in)  "<TurnLghtRight_D_Rq>"
  bus_selector/26 -> DrStatDrv_B_Actl/1(in)  "<DrStatDrv_B_Actl>"
  bus_selector/27 -> DrStatPsngr_B_Actl/1(in)  "<DrStatPsngr_B_Actl>"
  bus_selector/28 -> DrStatHood_B_Actl/1(in)  "<DrStatHood_B_Actl>"
  bus_selector/29 -> DrStatInnrTgate_B_Actl/1(in)  "<DrStatInnrTgate_B_Actl>"
  bus_selector/30 -> Delay_Accy/1(in)  "<Delay_Accy>"
  bus_selector/31 -> FogLghtFrontOn_B_Stat/1(in)  "<FogLghtFrontOn_B_Stat>"
  in/1 -> bus_selector/1

== system test_mdl_NI/CAN_Signal/BCM/Body_Info_10_0x3BA ==
  in : Inport
  GenericSwtch1_No_Actl : Subsystem
  GenericSwtch2_No_Actl : Subsystem
  GenericSwtch3_No_Actl : Subsystem
  bus_creator : BusCreator  Inputs=3
  bus_selector : BusSelector  OutputSignals=GenericSwtch1_No_Actl,GenericSwtch2_No_Actl,GenericSwtch3_No_Actl
  out_port : Outport
  wires:
  bus_creator/1 -> out_port/1  "Body_Info_10_0x3BA"
  GenericSwtch1_No_Actl/1(out) -> bus_creator/1  "GenericSwtch1_No_Actl"
  GenericSwtch2_No_Actl/1(out) -> bus_creator/2  "GenericSwtch2_No_Actl"
  GenericSwtch3_No_Actl/1(out) -> bus_creator/3  "GenericSwtch3_No_Actl"
  bus_selector/1 -> GenericSwtch1_No_Actl/1(in)  "<GenericSwtch1_No_Actl>"
  bus_selector/2 -> GenericSwtch2_No_Actl/1(in)  "<GenericSwtch2_No_Actl>"
  bus_selector/3 -> GenericSwtch3_No_Actl/1(in)  "<GenericSwtch3_No_Actl>"
  in/1 -> bus_selector/1

== system test_mdl_NI/CAN_Signal/BCM/Body_Info_12_0x26E ==
  in : Inport
  FobCtlPssvData_No_Actl : Subsystem
  FobCtlRollCode_No_Stat : Subsystem
  FobCtlType_D_Stat : Subsystem
  bus_creator : BusCreator  Inputs=3
  bus_selector : BusSelector  OutputSignals=FobCtlPssvData_No_Actl,FobCtlRollCode_No_Stat,FobCtlType_D_Stat
  out_port : Outport
  wires:
  bus_creator/1 -> out_port/1  "Body_Info_12_0x26E"
  FobCtlPssvData_No_Actl/1(out) -> bus_creator/1  "FobCtlPssvData_No_Actl"
  FobCtlRollCode_No_Stat/1(out) -> bus_creator/2  "FobCtlRollCode_No_Stat"
  FobCtlType_D_Stat/1(out) -> bus_creator/3  "FobCtlType_D_Stat"
  bus_selector/1 -> FobCtlPssvData_No_Actl/1(in)  "<FobCtlPssvData_No_Actl>"
  bus_selector/2 -> FobCtlRollCode_No_Stat/1(in)  "<FobCtlRollCode_No_Stat>"
  bus_selector/3 -> FobCtlType_D_Stat/1(in)  "<FobCtlType_D_Stat>"
  in/1 -> bus_selector/1

== system test_mdl_NI/CAN_Signal/BCM/Body_Info_4_0x242 ==
  in : Inport
  BattULo_I_Actl : Subsystem
  BattULo_U_Actl : Subsystem
  BrkTrnShifLck_B_Stat : Subsystem
  DcacElPw_D_Rq : Subsystem
  DriverCrankingReq : Subsystem
  EngOff_T_Actl : Subsystem
  FuelPumpPwr_D_Stat : Subsystem
  PrkLckCtlAvail_T_Stat : Subsystem
  PrkLckCtlMsgTxt_D_Rq : Subsystem
  PrkLckCtlTow_B_Enbl : Subsystem
  PrkLckCtlUnlck_D_Stat : Subsystem
  PrkLckCtl_B_Enbl : Subsystem
  PtLatchActv_B_RqBcm : Subsystem
  ReFuelSwtchStat_D_Actl : Subsystem
  bus_creator : BusCreator  Inputs=15
  bus_selector : BusSelector  OutputSignals=BattULo_I_Actl,BattULo_U_Actl,BrkTrnShifLck_B_Stat,DcacElPw_D_Rq,DriverCrankingReq,EngOff_T_Actl,FuelPumpPwr_D_Stat,PrkLckCtlAvail_T_Stat,PrkLckCtlMsgTxt_D_Rq,PrkLckCtlTow_B_Enbl,PrkLckCtlUnlck_D_Stat,PrkLckCtl_B_Enbl,PtLatchActv_B_RqBcm,ReFuelSwtchStat_D_Actl,immoSecureIdleMode
  immoSecureIdleMode : Subsystem
  out_port : Outport
  wires:
  bus_creator/1 -> out_port/1  "Body_Info_4_0x242"
  BattULo_I_Actl/1(out) -> bus_creator/1  "BattULo_I_Actl"
  BattULo_U_Actl/1(out) -> bus_creator/2  "BattULo_U_Actl"
  BrkTrnShifLck_B_Stat/1(out) -> bus_creator/3  "BrkTrnShifLck_B_Stat"
  DcacElPw_D_Rq/1(out) -> bus_creator/4  "DcacElPw_D_Rq"
  DriverCrankingReq/1(out) -> bus_creator/5  "DriverCrankingReq"
  EngOff_T_Actl/1(out) -> bus_creator/6  "EngOff_T_Actl"
  FuelPumpPwr_D_Stat/1(out) -> bus_creator/7  "FuelPumpPwr_D_Stat"
  PrkLckCtlAvail_T_Stat/1(out) -> bus_creator/8  "PrkLckCtlAvail_T_Stat"
  PrkLckCtlMsgTxt_D_Rq/1(out) -> bus_creator/9  "PrkLckCtlMsgTxt_D_Rq"
  PrkLckCtlTow_B_Enbl/1(out) -> bus_creator/10  "PrkLckCtlTow_B_Enbl"
  PrkLckCtlUnlck_D_Stat/1(out) -> bus_creator/11  "PrkLckCtlUnlck_D_Stat"
  PrkLckCtl_B_Enbl/1(out) -> bus_creator/12  "PrkLckCtl_B_Enbl"
  PtLatchActv_B_RqBcm/1(out) -> bus_creator/13  "PtLatchActv_B_RqBcm"
  ReFuelSwtchStat_D_Actl/1(out) -> bus_creator/14  "ReFuelSwtchStat_D_Actl"
  immoSecureIdleMode/1(out) -> bus_creator/15  "immoSecureIdleMode"
  bus_selector/1 -> BattULo_I_Actl/1(in)  "<BattULo_I_Actl>"
  bus_selector/2 -> BattULo_U_Actl/1(in)  "<BattULo_U_Actl>"
  bus_selector/3 -> BrkTrnShifLck_B_Stat/1(in)  "<BrkTrnShifLck_B_Stat>"
  bus_selector/4 -> DcacElPw_D_Rq/1(in)  "<DcacElPw_D_Rq>"
  bus_selector/5 -> DriverCrankingReq/1(in)  "<DriverCrankingReq>"
  bus_selector/6 -> EngOff_T_Actl/1(in)  "<EngOff_T_Actl>"
  bus_selector/7 -> FuelPumpPwr_D_Stat/1(in)  "<FuelPumpPwr_D_Stat>"
  bus_selector/8 -> PrkLckCtlAvail_T_Stat/1(in)  "<PrkLckCtlAvail_T_Stat>"
  bus_selector/9 -> PrkLckCtlMsgTxt_D_Rq/1(in)  "<PrkLckCtlMsgTxt_D_Rq>"
  bus_selector/10 -> PrkLckCtlTow_B_Enbl/1(in)  "<PrkLckCtlTow_B_Enbl>"
  bus_selector/11 -> PrkLckCtlUnlck_D_Stat/1(in)  "<PrkLckCtlUnlck_D_Stat>"
  bus_selector/12 -> PrkLckCtl_B_Enbl/1(in)  "<PrkLckCtl_B_Enbl>"
  bus_selector/13 -> PtLatchActv_B_RqBcm/1(in)  "<PtLatchActv_B_RqBcm>"
  bus_selector/14 -> ReFuelSwtchStat_D_Actl/1(in)  "<ReFuelSwtchStat_D_Actl>"
  bus_selector/15 -> immoSecureIdleMode/1(in)  "<immoSecureIdleMode>"
  in/1 -> bus_selector/1

== system test_mdl_NI/CAN_Signal/BCM/Body_Info_6_0x38D ==
  in : Inport
  DrLatchMsgTxt_D_Rq : Subsystem
  ElPwPoint_D_Rq : Subsystem
  HeadLghtHiPrmsn_D_Stat : Subsystem
  IgnPsswrdDsply_B_Rq : Subsystem
  KeyAdmnTot_No_Cnt : Subsystem
  KeyMykeyTot_No_Cnt : Subsystem
  Keycode_Status : Subsystem
  PEBackupSlot_Stats : Subsystem
  PoliceIdlMde_D_Stat : Subsystem
  PrmtrAlrmEvnt_D_Stat : Subsystem
  PrsnlDevcChrgEnbl_B_Rq : Subsystem
  SecurityMsgTxt_D_Rq : Subsystem
  SteWhlLckMsgTxt_D_Rq : Subsystem
  TracKeyMde_D_Stat : Subsystem
  bus_creator : BusCreator  Inputs=15
  bus_selector : BusSelector  OutputSignals=KeyAdmnTot_No_Cnt,KeyMykeyTot_No_Cnt,Keycode_Status,PEBackupSlot_Stats,SteWhlLckMsgTxt_D_Rq,immoMsgTxt_D_Rq,PrmtrAlrmEvnt_D_Stat,SecurityMsgTxt_D_Rq,TracKeyMde_D_Stat,DrLatchMsgTxt_D_Rq,PrsnlDevcChrgEnbl_B_Rq,PoliceIdlMde_D_Stat,HeadLghtHiPrmsn_D_Stat,ElPwPoint_D_Rq,IgnPsswrdDsply_B_Rq
  immoMsgTxt_D_Rq : Subsystem
  out_port : Outport
  wires:
  bus_creator/1 -> out_port/1  "Body_Info_6_0x38D"
  KeyAdmnTot_No_Cnt/1(out) -> bus_creator/1  "KeyAdmnTot_No_Cnt"
  KeyMykeyTot_No_Cnt/1(out) -> bus_creator/2  "KeyMykeyTot_No_Cnt"
  Keycode_Status/1(out) -> bus_creator/3  "Keycode_Status"
  PEBackupSlot_Stats/1(out) -> bus_creator/4  "PEBackupSlot_Stats"
  SteWhlLckMsgTxt_D_Rq/1(out) -> bus_creator/5  "SteWhlLckMsgTxt_D_Rq"
  immoMsgTxt_D_Rq/1(out) -> bus_creator/6  "immoMsgTxt_D_Rq"
  PrmtrAlrmEvnt_D_Stat/1(out) -> bus_creator/7  "PrmtrAlrmEvnt_D_Stat"
  SecurityMsgTxt_D_Rq/1(out) -> bus_creator/8  "SecurityMsgTxt_D_Rq"
  TracKeyMde_D_Stat/1(out) -> bus_creator/9  "TracKeyMde_D_Stat"
  DrLatchMsgTxt_D_Rq/1(out) -> bus_creator/10  "DrLatchMsgTxt_D_Rq"
  PrsnlDevcChrgEnbl_B_Rq/1(out) -> bus_creator/11  "PrsnlDevcChrgEnbl_B_Rq"
  PoliceIdlMde_D_Stat/1(out) -> bus_creator/12  "PoliceIdlMde_D_Stat"
  HeadLghtHiPrmsn_D_Stat/1(out) -> bus_creator/13  "HeadLghtHiPrmsn_D_Stat"
  ElPwPoint_D_Rq/1(out) -> bus_creator/14  "ElPwPoint_D_Rq"
  IgnPsswrdDsply_B_Rq/1(out) -> bus_creator/15  "IgnPsswrdDsply_B_Rq"
  bus_selector/1 -> KeyAdmnTot_No_Cnt/1(in)  "<KeyAdmnTot_No_Cnt>"
  bus_selector/2 -> KeyMykeyTot_No_Cnt/1(in)  "<KeyMykeyTot_No_Cnt>"
  bus_selector/3 -> Keycode_Status/1(in)  "<Keycode_Status>"
  bus_selector/4 -> PEBackupSlot_Stats/1(in)  "<PEBackupSlot_Stats>"
  bus_selector/5 -> SteWhlLckMsgTxt_D_Rq/1(in)  "<SteWhlLckMsgTxt_D_Rq>"
  bus_selector/6 -> immoMsgTxt_D_Rq/1(in)  "<immoMsgTxt_D_Rq>"
  bus_selector/7 -> PrmtrAlrmEvnt_D_Stat/1(in)  "<PrmtrAlrmEvnt_D_Stat>"
  bus_selector/8 -> SecurityMsgTxt_D_Rq/1(in)  "<SecurityMsgTxt_D_Rq>"
  bus_selector/9 -> TracKeyMde_D_Stat/1(in)  "<TracKeyMde_D_Stat>"
  bus_selector/10 -> DrLatchMsgTxt_D_Rq/1(in)  "<DrLatchMsgTxt_D_Rq>"
  bus_selector/11 -> PrsnlDevcChrgEnbl_B_Rq/1(in)  "<PrsnlDevcChrgEnbl_B_Rq>"
  bus_selector/12 -> PoliceIdlMde_D_Stat/1(in)  "<PoliceIdlMde_D_Stat>"
  bus_selector/13 -> HeadLghtHiPrmsn_D_Stat/1(in)  "<HeadLghtHiPrmsn_D_Stat>"
  bus_selector/14 -> ElPwPoint_D_Rq/1(in)  "<ElPwPoint_D_Rq>"
  bus_selector/15 -> IgnPsswrdDsply_B_Rq/1(in)  "<IgnPsswrdDsply_B_Rq>"
  in/1 -> bus_selector/1

== system test_mdl_NI/CAN_Signal/BCM/Body_Info_7_0x3B1 ==
  in : Inport
  KeyOffMde_D_Actl : Subsystem
  bus_creator : BusCreator  Inputs=1
  bus_selector : BusSelector  OutputSignals=KeyOffMde_D_Actl
  out_port : Outport
  wires:
  bus_creator/1 -> out_port/1  "Body_Info_7_0x3B1"
  KeyOffMde_D_Actl/1(out) -> bus_creator/1  "KeyOffMde_D_Actl"
  bus_selector/1 -> KeyOffMde_D_Actl/1(in)  "<KeyOffMde_D_Actl>"
  in/1 -> bus_selector/1

== system test_mdl_NI/CAN_Signal/BCM/Body_Info_8_0x3B9 ==
  in : Inport
  ChrgCordLck_B_Stat : Subsystem
  ChrgCordResp1_No_Actl : Subsystem
  ChrgCordResp2_No_Actl : Subsystem
  WakeAlarm0_D_Stat : Subsystem
  WakeAlarm1_D_Stat : Subsystem
  WakeAlarm2_D_Stat : Subsystem
  WakeAlarm3_D_Stat : Subsystem
  bus_creator : BusCreator  Inputs=7
  bus_selector : BusSelector  OutputSignals=WakeAlarm0_D_Stat,WakeAlarm1_D_Stat,WakeAlarm2_D_Stat,WakeAlarm3_D_Stat,ChrgCordResp1_No_Actl,ChrgCordResp2_No_Actl,ChrgCordLck_B_Stat
  out_port : Outport
  wires:
  bus_creator/1 -> out_port/1  "Body_Info_8_0x3B9"
  WakeAlarm0_D_Stat/1(out) -> bus_creator/1  "WakeAlarm0_D_Stat"
  WakeAlarm1_D_Stat/1(out) -> bus_creator/2  "WakeAlarm1_D_Stat"
  WakeAlarm2_D_Stat/1(out) -> bus_creator/3  "WakeAlarm2_D_Stat"
  WakeAlarm3_D_Stat/1(out) -> bus_creator/4  "WakeAlarm3_D_Stat"
  ChrgCordResp1_No_Actl/1(out) -> bus_creator/5  "ChrgCordResp1_No_Actl"
  ChrgCordResp2_No_Actl/1(out) -> bus_creator/6  "ChrgCordResp2_No_Actl"
  ChrgCordLck_B_Stat/1(out) -> bus_creator/7  "ChrgCordLck_B_Stat"
  bus_selector/1 -> WakeAlarm0_D_Stat/1(in)  "<WakeAlarm0_D_Stat>"
  bus_selector/2 -> WakeAlarm1_D_Stat/1(in)  "<WakeAlarm1_D_Stat>"
  bus_selector/3 -> WakeAlarm2_D_Stat/1(in)  "<WakeAlarm2_D_Stat>"
  bus_selector/4 -> WakeAlarm3_D_Stat/1(in)  "<WakeAlarm3_D_Stat>"
  bus_selector/5 -> ChrgCordResp1_No_Actl/1(in)  "<ChrgCordResp1_No_Actl>"
  bus_selector/6 -> ChrgCordResp2_No_Actl/1(in)  "<ChrgCordResp2_No_Actl>"
  bus_selector/7 -> ChrgCordLck_B_Stat/1(in)  "<ChrgCordLck_B_Stat>"
  in/1 -> bus_selector/1

== system test_mdl_NI/CAN_Signal/BCM/Body_Info_9_0x3A3 ==
  in : Inport
  AdvStrt_D_Stat : Subsystem
  CrnkInhbt_B_Stat : Subsystem
  CrnkInhbt_No_Cnt : Subsystem
  CrnkInhbt_No_Cs : Subsystem
  DrvInCtl_B_Stat : Subsystem
  EngStrtActv_B_Stat : Subsystem
  EngStrt_B_Rq : Subsystem
  IgnPreOffActv_B_Stat : Subsystem
  StrtrMtrCtlDStat_No_Cs : Subsystem
  VehOnSrc_D_Stat : Subsystem
  bus_creator : BusCreator  Inputs=10
  bus_selector : BusSelector  OutputSignals=CrnkInhbt_B_Stat,CrnkInhbt_No_Cnt,IgnPreOffActv_B_Stat,DrvInCtl_B_Stat,EngStrt_B_Rq,CrnkInhbt_No_Cs,AdvStrt_D_Stat,VehOnSrc_D_Stat,StrtrMtrCtlDStat_No_Cs,EngStrtActv_B_Stat
  out_port : Outport
  wires:
  bus_creator/1 -> out_port/1  "Body_Info_9_0x3A3"
  CrnkInhbt_B_Stat/1(out) -> bus_creator/1  "CrnkInhbt_B_Stat"
  CrnkInhbt_No_Cnt/1(out) -> bus_creator/2  "CrnkInhbt_No_Cnt"
  IgnPreOffActv_B_Stat/1(out) -> bus_creator/3  "IgnPreOffActv_B_Stat"
  DrvInCtl_B_Stat/1(out) -> bus_creator/4  "DrvInCtl_B_Stat"
  EngStrt_B_Rq/1(out) -> bus_creator/5  "EngStrt_B_Rq"
  CrnkInhbt_No_Cs/1(out) -> bus_creator/6  "CrnkInhbt_No_Cs"
  AdvStrt_D_Stat/1(out) -> bus_creator/7  "AdvStrt_D_Stat"
  VehOnSrc_D_Stat/1(out) -> bus_creator/8  "VehOnSrc_D_Stat"
  StrtrMtrCtlDStat_No_Cs/1(out) -> bus_creator/9  "StrtrMtrCtlDStat_No_Cs"
  EngStrtActv_B_Stat/1(out) -> bus_creator/10  "EngStrtActv_B_Stat"
  bus_selector/1 -> CrnkInhbt_B_Stat/1(in)  "<CrnkInhbt_B_Stat>"
  bus_selector/2 -> CrnkInhbt_No_Cnt/1(in)  "<CrnkInhbt_No_Cnt>"
  bus_selector/3 -> IgnPreOffActv_B_Stat/1(in)  "<IgnPreOffActv_B_Stat>"
  bus_selector/4 -> DrvInCtl_B_Stat/1(in)  "<DrvInCtl_B_Stat>"
  bus_selector/5 -> EngStrt_B_Rq/1(in)  "<EngStrt_B_Rq>"
  bus_selector/6 -> CrnkInhbt_No_Cs/1(in)  "<CrnkInhbt_No_Cs>"
  bus_selector/7 -> AdvStrt_D_Stat/1(in)  "<AdvStrt_D_Stat>"
  bus_selector/8 -> VehOnSrc_D_Stat/1(in)  "<VehOnSrc_D_Stat>"
  bus_selector/9 -> StrtrMtrCtlDStat_No_Cs/1(in)  "<StrtrMtrCtlDStat_No_Cs>"
  bus_selector/10 -> EngStrtActv_B_Stat/1(in)  "<EngStrtActv_B_Stat>"
  in/1 -> bus_selector/1

== system test_mdl_NI/CAN_Signal/BCM/CMPS_FDM_Info_Status_0x3C7 ==
  in : Inport
  CamPDCGuidStat : Subsystem
  CamZoomActiveState : Subsystem
  CamraOvrlDyn_D_Actl : Subsystem
  CamraOvrlStat_D_Actl : Subsystem
  CamraOvrlTow_D_Actl : Subsystem
  CamraViewSplit_D_Actl : Subsystem
  CamraZoomMan_D_Actl : Subsystem
  bus_creator : BusCreator  Inputs=7
  bus_selector : BusSelector  OutputSignals=CamraViewSplit_D_Actl,CamraOvrlDyn_D_Actl,CamraZoomMan_D_Actl,CamPDCGuidStat,CamZoomActiveState,CamraOvrlStat_D_Actl,CamraOvrlTow_D_Actl
  out_port : Outport
  wires:
  bus_creator/1 -> out_port/1  "CMPS_FDM_Info_Status_0x3C7"
  CamraViewSplit_D_Actl/1(out) -> bus_creator/1  "CamraViewSplit_D_Actl"
  CamraOvrlDyn_D_Actl/1(out) -> bus_creator/2  "CamraOvrlDyn_D_Actl"
  CamraZoomMan_D_Actl/1(out) -> bus_creator/3  "CamraZoomMan_D_Actl"
  CamPDCGuidStat/1(out) -> bus_creator/4  "CamPDCGuidStat"
  CamZoomActiveState/1(out) -> bus_creator/5  "CamZoomActiveState"
  CamraOvrlStat_D_Actl/1(out) -> bus_creator/6  "CamraOvrlStat_D_Actl"
  CamraOvrlTow_D_Actl/1(out) -> bus_creator/7  "CamraOvrlTow_D_Actl"
  bus_selector/1 -> CamraViewSplit_D_Actl/1(in)  "<CamraViewSplit_D_Actl>"
  bus_selector/2 -> CamraOvrlDyn_D_Actl/1(in)  "<CamraOvrlDyn_D_Actl>"
  bus_selector/3 -> CamraZoomMan_D_Actl/1(in)  "<CamraZoomMan_D_Actl>"
  bus_selector/4 -> CamPDCGuidStat/1(in)  "<CamPDCGuidStat>"
  bus_selector/5 -> CamZoomActiveState/1(in)  "<CamZoomActiveState>"
  bus_selector/6 -> CamraOvrlStat_D_Actl/1(in)  "<CamraOvrlStat_D_Actl>"
  bus_selector/7 -> CamraOvrlTow_D_Actl/1(in)  "<CamraOvrlTow_D_Actl>"
  in/1 -> bus_selector/1

== system test_mdl_NI/CAN_Signal/BCM/CellPhonePassport_Stat_1_0x447 ==
  in : Inport
  HeadLghtOn_D_Rq : Subsystem
  KeyProg_No_Actl : Subsystem
  PepsKeyActv_D_Stat : Subsystem
  PepsKeyFound_No_Actl : Subsystem
  Pers1Phone_D_Stat : Subsystem
  Pers2Phone_D_Stat : Subsystem
  Pers3Phone_D_Stat : Subsystem
  Pers4Phone_D_Stat : Subsystem
  RstrtSetting_T_Actl : Subsystem
  Rstrt_T_Actl : Subsystem
  VehLck_D_Dsply : Subsystem
  bus_creator : BusCreator  Inputs=11
  bus_selector : BusSelector  OutputSignals=KeyProg_No_Actl,PepsKeyActv_D_Stat,Rstrt_T_Actl,RstrtSetting_T_Actl,PepsKeyFound_No_Actl,HeadLghtOn_D_Rq,VehLck_D_Dsply,Pers1Phone_D_Stat,Pers2Phone_D_Stat,Pers3Phone_D_Stat,Pers4Phone_D_Stat
  out_port : Outport
  wires:
  bus_creator/1 -> out_port/1  "CellPhonePassport_Stat_1_0x447"
  KeyProg_No_Actl/1(out) -> bus_creator/1  "KeyProg_No_Actl"
  PepsKeyActv_D_Stat/1(out) -> bus_creator/2  "PepsKeyActv_D_Stat"
  Rstrt_T_Actl/1(out) -> bus_creator/3  "Rstrt_T_Actl"
  RstrtSetting_T_Actl/1(out) -> bus_creator/4  "RstrtSetting_T_Actl"
  PepsKeyFound_No_Actl/1(out) -> bus_creator/5  "PepsKeyFound_No_Actl"
  HeadLghtOn_D_Rq/1(out) -> bus_creator/6  "HeadLghtOn_D_Rq"
  VehLck_D_Dsply/1(out) -> bus_creator/7  "VehLck_D_Dsply"
  Pers1Phone_D_Stat/1(out) -> bus_creator/8  "Pers1Phone_D_Stat"
  Pers2Phone_D_Stat/1(out) -> bus_creator/9  "Pers2Phone_D_Stat"
  Pers3Phone_D_Stat/1(out) -> bus_creator/10  "Pers3Phone_D_Stat"
  Pers4Phone_D_Stat/1(out) -> bus_creator/11  "Pers4Phone_D_Stat"
  bus_selector/1 -> KeyProg_No_Actl/1(in)  "<KeyProg_No_Actl>"
  bus_selector/2 -> PepsKeyActv_D_Stat/1(in)  "<PepsKeyActv_D_Stat>"
  bus_selector/3 -> Rstrt_T_Actl/1(in)  "<Rstrt_T_Actl>"
  bus_selector/4 -> RstrtSetting_T_Actl/1(in)  "<RstrtSetting_T_Actl>"
  bus_selector/5 -> PepsKeyFound_No_Actl/1(in)  "<PepsKeyFound_No_Actl>"
  bus_selector/6 -> HeadLghtOn_D_Rq/1(in)  "<HeadLghtOn_D_Rq>"
  bus_selector/7 -> VehLck_D_Dsply/1(in)  "<VehLck_D_Dsply>"
  bus_selector/8 -> Pers1Phone_D_Stat/1(in)  "<Pers1Phone_D_Stat>"
  bus_selector/9 -> Pers2Phone_D_Stat/1(in)  "<Pers2Phone_D_Stat>"
  bus_selector/10 -> Pers3Phone_D_Stat/1(in)  "<Pers3Phone_D_Stat>"
  bus_selector/11 -> Pers4Phone_D_Stat/1(in)  "<Pers4Phone_D_Stat>"
  in/1 -> bus_selector/1

== system test_mdl_NI/CAN_Signal/BCM/GGCC_Config_Mgmt_ID_1_0x40A ==
  in : Inport
  VehicleGGCCData : Subsystem
  bus_creator : BusCreator  Inputs=1
  bus_selector : BusSelector  OutputSignals=VehicleGGCCData
  out_port : Outport
  wires:
  bus_creator/1 -> out_port/1  "GGCC_Config_Mgmt_ID_1_0x40A"
  VehicleGGCCData/1(out) -> bus_creator/1  "VehicleGGCCData"
  bus_selector/1 -> VehicleGGCCData/1(in)  "<VehicleGGCCData>"
  in/1 -> bus_selector/1

== system test_mdl_NI/CAN_Signal/BCM/GlobalClock_Data_0x84 ==
  in : Inport
  GlblClkDay_No_Actl : Subsystem
  GlblClkHr_No_Actl : Subsystem
  GlblClkMnte_No_Actl : Subsystem
  GlblClkScnd_No_Actl : Subsystem
  GlblClkYr_No_Actl : Subsystem
  bus_creator : BusCreator  Inputs=5
  bus_selector : BusSelector  OutputSignals=GlblClkYr_No_Actl,GlblClkDay_No_Actl,GlblClkMnte_No_Actl,GlblClkScnd_No_Actl,GlblClkHr_No_Actl
  out_port : Outport
  wires:
  bus_creator/1 -> out_port/1  "GlobalClock_Data_0x84"
  GlblClkYr_No_Actl/1(out) -> bus_creator/1  "GlblClkYr_No_Actl"
  GlblClkDay_No_Actl/1(out) -> bus_creator/2  "GlblClkDay_No_Actl"
  GlblClkMnte_No_Actl/1(out) -> bus_creator/3  "GlblClkMnte_No_Actl"
  GlblClkScnd_No_Actl/1(out) -> bus_creator/4  "GlblClkScnd_No_Actl"
  GlblClkHr_No_Actl/1(out) -> bus_creator/5  "GlblClkHr_No_Actl"
  bus_selector/1 -> GlblClkYr_No_Actl/1(in)  "<GlblClkYr_No_Actl>"
  bus_selector/2 -> GlblClkDay_No_Actl/1(in)  "<GlblClkDay_No_Actl>"
  bus_selector/3 -> GlblClkMnte_No_Actl/1(in)  "<GlblClkMnte_No_Actl>"
  bus_selector/4 -> GlblClkScnd_No_Actl/1(in)  "<GlblClkScnd_No_Actl>"
  bus_selector/5 -> GlblClkHr_No_Actl/1(in)  "<GlblClkHr_No_Actl>"
  in/1 -> bus_selector/1

== system test_mdl_NI/CAN_Signal/BCM/Global_PATS_Control_Info2_0x42 ==
  in : Inport
  bus_creator : BusCreator  Inputs=2
  bus_selector : BusSelector  OutputSignals=immoControlCmd_T2,immoControlData_T2
  immoControlCmd_T2 : Subsystem
  immoControlData_T2 : Subsystem
  out_port : Outport
  wires:
  bus_creator/1 -> out_port/1  "Global_PATS_Control_Info2_0x42"
  immoControlCmd_T2/1(out) -> bus_creator/1  "immoControlCmd_T2"
  immoControlData_T2/1(out) -> bus_creator/2  "immoControlData_T2"
  bus_selector/1 -> immoControlCmd_T2/1(in)  "<immoControlCmd_T2>"
  bus_selector/2 -> immoControlData_T2/1(in)  "<immoControlData_T2>"
  in/1 -> bus_selector/1

== system test_mdl_NI/CAN_Signal/BCM/Global_PATS_Control_Info_0x41 ==
  in : Inport
  bus_creator : BusCreator  Inputs=2
  bus_selector : BusSelector  OutputSignals=immoControlCmd_T1,immoControlData_T1
  immoControlCmd_T1 : Subsystem
  immoControlData_T1 : Subsystem
  out_port : Outport
  wires:
  bus_creator/1 -> out_port/1  "Global_PATS_Control_Info_0x41"
  immoControlCmd_T1/1(out) -> bus_creator/1  "immoControlCmd_T1"
  immoControlData_T1/1(out) -> bus_creator/2  "immoControlData_T1"
  bus_selector/1 -> immoControlCmd_T1/1(in)  "<immoControlCmd_T1>"
  bus_selector/2 -> immoControlData_T1/1(in)  "<immoControlData_T1>"
  in/1 -> bus_selector/1

== system test_mdl_NI/CAN_Signal/BCM/Locking_Systems_2_0x331 ==
  in : Inport
  ChildLckMde_B_Stat : Subsystem
  ChildLck_D_Dsply : Subsystem
  DrTgateExtSwMde_B_Stat : Subsystem
  DrTgateOpen_B_Rq : Subsystem
  FobComm_D_Stat : Subsystem
  Keyfob_Pad_Msg_Count : Subsystem
  L_Pwr_Sliding_Dr_Rqst : Subsystem
  LockInhibit : Subsystem
  Lockmsgtxt_D_Rq : Subsystem
  Power_Decklid_Rqst : Subsystem
  Power_Liftgate_Rqst : Subsystem
  R_Pwr_Sliding_Dr_Rqst : Subsystem
  Remote_Device_Feedback : Subsystem
  RollCodeUnlock : Subsystem
  VehLckInd_D_Rq : Subsystem
  Veh_Lock_EvNum : Subsystem
  Veh_Lock_Requestor : Subsystem
  Veh_Lock_Status : Subsystem
  Veh_Lock_Sub_Id : Subsystem
  WindowLockout_B_Stat : Subsystem
  bus_creator : BusCreator  Inputs=20
  bus_selector : BusSelector  OutputSignals=ChildLck_D_Dsply,FobComm_D_Stat,L_Pwr_Sliding_Dr_Rqst,LockInhibit,Power_Decklid_Rqst,Power_Liftgate_Rqst,Keyfob_Pad_Msg_Count,RollCodeUnlock,Lockmsgtxt_D_Rq,R_Pwr_Sliding_Dr_Rqst,WindowLockout_B_Stat,Veh_Lock_Status,DrTgateExtSwMde_B_Stat,Veh_Lock_EvNum,Veh_Lock_Requestor,Remote_Device_Feedback,Veh_Lock_Sub_Id,DrTgateOpen_B_Rq,VehLckInd_D_Rq,ChildLckMde_B_Stat
  out_port : Outport
  wires:
  bus_creator/1 -> out_port/1  "Locking_Systems_2_0x331"
  ChildLck_D_Dsply/1(out) -> bus_creator/1  "ChildLck_D_Dsply"
  FobComm_D_Stat/1(out) -> bus_creator/2  "FobComm_D_Stat"
  L_Pwr_Sliding_Dr_Rqst/1(out) -> bus_creator/3  "L_Pwr_Sliding_Dr_Rqst"
  LockInhibit/1(out) -> bus_creator/4  "LockInhibit"
  Power_Decklid_Rqst/1(out) -> bus_creator/5  "Power_Decklid_Rqst"
  Power_Liftgate_Rqst/1(out) -> bus_creator/6  "Power_Liftgate_Rqst"
  Keyfob_Pad_Msg_Count/1(out) -> bus_creator/7  "Keyfob_Pad_Msg_Count"
  RollCodeUnlock/1(out) -> bus_creator/8  "RollCodeUnlock"
  Lockmsgtxt_D_Rq/1(out) -> bus_creator/9  "Lockmsgtxt_D_Rq"
  R_Pwr_Sliding_Dr_Rqst/1(out) -> bus_creator/10  "R_Pwr_Sliding_Dr_Rqst"
  WindowLockout_B_Stat/1(out) -> bus_creator/11  "WindowLockout_B_Stat"
  Veh_Lock_Status/1(out) -> bus_creator/12  "Veh_Lock_Status"
  DrTgateExtSwMde_B_Stat/1(out) -> bus_creator/13  "DrTgateExtSwMde_B_Stat"
  Veh_Lock_EvNum/1(out) -> bus_creator/14  "Veh_Lock_EvNum"
  Veh_Lock_Requestor/1(out) -> bus_creator/15  "Veh_Lock_Requestor"
  Remote_Device_Feedback/1(out) -> bus_creator/16  "Remote_Device_Feedback"
  Veh_Lock_Sub_Id/1(out) -> bus_creator/17  "Veh_Lock_Sub_Id"
  DrTgateOpen_B_Rq/1(out) -> bus_creator/18  "DrTgateOpen_B_Rq"
  VehLckInd_D_Rq/1(out) -> bus_creator/19  "VehLckInd_D_Rq"
  ChildLckMde_B_Stat/1(out) -> bus_creator/20  "ChildLckMde_B_Stat"
  bus_selector/1 -> ChildLck_D_Dsply/1(in)  "<ChildLck_D_Dsply>"
  bus_selector/2 -> FobComm_D_Stat/1(in)  "<FobComm_D_Stat>"
  bus_selector/3 -> L_Pwr_Sliding_Dr_Rqst/1(in)  "<L_Pwr_Sliding_Dr_Rqst>"
  bus_selector/4 -> LockInhibit/1(in)  "<LockInhibit>"
  bus_selector/5 -> Power_Decklid_Rqst/1(in)  "<Power_Decklid_Rqst>"
  bus_selector/6 -> Power_Liftgate_Rqst/1(in)  "<Power_Liftgate_Rqst>"
  bus_selector/7 -> Keyfob_Pad_Msg_Count/1(in)  "<Keyfob_Pad_Msg_Count>"
  bus_selector/8 -> RollCodeUnlock/1(in)  "<RollCodeUnlock>"
  bus_selector/9 -> Lockmsgtxt_D_Rq/1(in)  "<Lockmsgtxt_D_Rq>"
  bus_selector/10 -> R_Pwr_Sliding_Dr_Rqst/1(in)  "<R_Pwr_Sliding_Dr_Rqst>"
  bus_selector/11 -> WindowLockout_B_Stat/1(in)  "<WindowLockout_B_Stat>"
  bus_selector/12 -> Veh_Lock_Status/1(in)  "<Veh_Lock_Status>"
  bus_selector/13 -> DrTgateExtSwMde_B_Stat/1(in)  "<DrTgateExtSwMde_B_Stat>"
  bus_selector/14 -> Veh_Lock_EvNum/1(in)  "<Veh_Lock_EvNum>"
  bus_selector/15 -> Veh_Lock_Requestor/1(in)  "<Veh_Lock_Requestor>"
  bus_selector/16 -> Remote_Device_Feedback/1(in)  "<Remote_Device_Feedback>"
  bus_selector/17 -> Veh_Lock_Sub_Id/1(in)  "<Veh_Lock_Sub_Id>"
  bus_selector/18 -> DrTgateOpen_B_Rq/1(in)  "<DrTgateOpen_B_Rq>"
  bus_selector/19 -> VehLckInd_D_Rq/1(in)  "<VehLckInd_D_Rq>"
  bus_selector/20 -> ChildLckMde_B_Stat/1(in)  "<ChildLckMde_B_Stat>"
  in/1 -> bus_selector/1
